simulink model "q2_b"  (R2016a)
settings: Solver=VariableStepAuto  SolverMode=SingleTasking  StartTime=0.0  StopTime=15  RelTol=1e-3
settings Model: Creator=pc  LastModifiedBy=pc
settings DataIOCC: LimitDataPoints=on  SaveOutput=off  SaveTime=off
settings OptimizationCC: BlockReduction=off  BooleanDataType=off
settings DebuggingCC: SaveWithParameterizedLinksMsg=none  UnderspecifiedInitializationDetection=Classic  MergeDetectMultiDrivingBlocksExec=none  SignalResolutionControl=TryResolveAllWithWarning  AllowSymbolicDim=off
settings HardwareCC: TargetUnknown=on

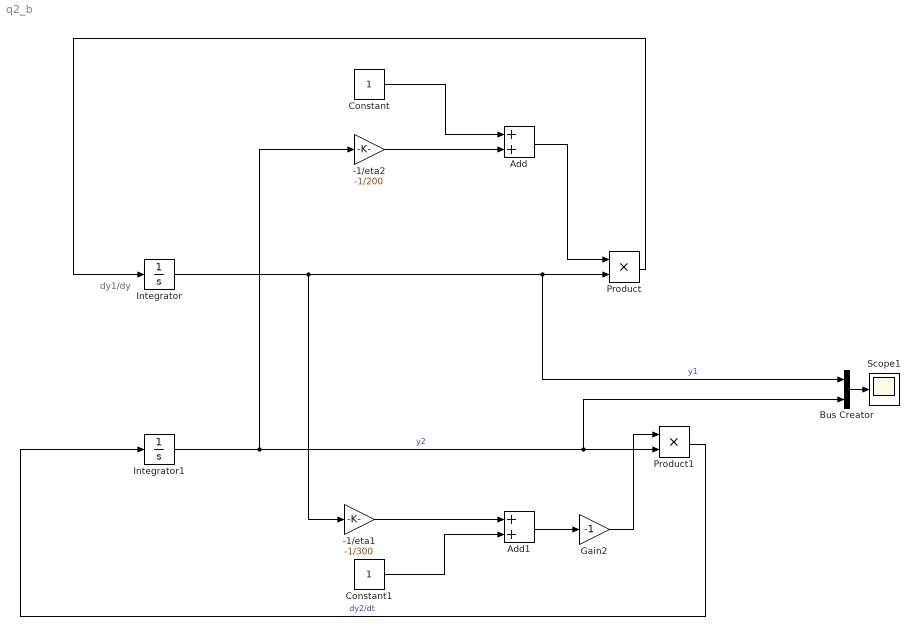
== system q2_b ==
  note: dy1/dy
  -1/eta1 : Gain  Gain=-1/300
  -1/eta2 : Gain  Gain=-1/200
  Add : Sum
  Add1 : Sum
  Bus Creator : BusCreator  Inputs=2
  Constant : Constant
  Constant1 : Constant
  Gain2 : Gain  Gain=-1
  Integrator : Integrator  InitialCondition=302
  Integrator1 : Integrator  InitialCondition=202
  Product : Product
  Product1 : Product
  Scope1 : Scope
  wires:
  Product/1 -> Integrator/1
  Integrator/1 -> -1/eta1/1, Bus Creator/1, Product/2  "y1"
  Integrator1/1 -> -1/eta2/1, Bus Creator/2, Product1/2  "y2"
  -1/eta2/1 -> Add/2
  Constant/1 -> Add/1
  Add/1 -> Product/1
  -1/eta1/1 -> Add1/1
  Constant1/1 -> Add1/2
  Add1/1 -> Gain2/1
  Gain2/1 -> Product1/1
  Product1/1 -> Integrator1/1  "dy2/dt"
  Bus Creator/1 -> Scope1/1
